simulink model "pd_controller"  (R2022a)
settings: Solver=VariableStepAuto  StartTime=0.0  StopTime=10.0  RelTol=1e-3
settings Model: Creator=Laptop-Academy.com  LastModifiedBy=Laptop-Academy.com

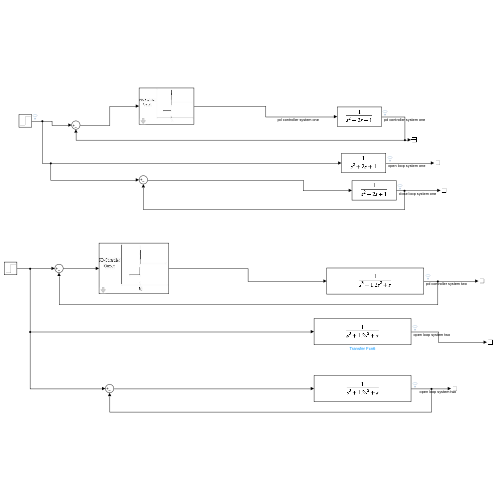
[thumbnail: Simulink's stored preview of the top-level diagram]
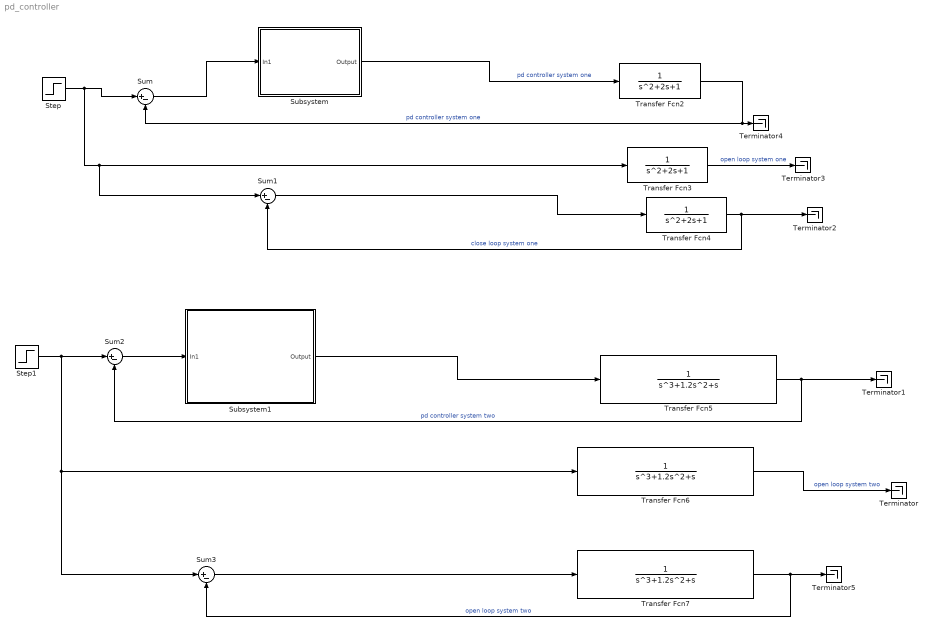
== system pd_controller ==
  Step : Step  SampleTime=0
  Step1 : Step  SampleTime=0
  Subsystem : Subsystem  mask{p=0, d=0}
      mask prompts: p "propotional gain (p)"; d "derivative gain (d)"
      mask Display: image("F:\os_academy_labs\pid_controller\media\pd.jpg")
  Subsystem1 : Subsystem  mask{p=0, d=0}
      mask prompts: p "proportional gain (p)"; d "derivartive gain (d)"
      mask Display: image("F:\os_academy_labs\pid_controller\media\pd.jpg")
  Sum{,1..3} (4 alike) : Sum  Inputs=|+-
  Terminator{,1..5} (6 alike) : Terminator
  Transfer Fcn2 : TransferFcn
  Transfer Fcn3 : TransferFcn
  Transfer Fcn4 : TransferFcn
  Transfer Fcn5 : TransferFcn  Denominator=[1 1.2 1 0]
  Transfer Fcn6 : TransferFcn  Denominator=[1 1.2 1 0]
  Transfer Fcn7 : TransferFcn  Denominator=[1 1.2 1 0]
  wires:
  Subsystem1/1(Output) -> Transfer Fcn5/1
  Transfer Fcn4/1 -> Sum1/2, Terminator2/1  "close loop system one"
  Transfer Fcn3/1 -> Terminator3/1  "open loop system one"
  Transfer Fcn2/1 -> Sum/2, Terminator4/1  "pd controller system one"
  Transfer Fcn6/1 -> Terminator/1  "open loop system two"
  Transfer Fcn7/1 -> Sum3/2, Terminator5/1  "open loop system two"
  Subsystem/1(Output) -> Transfer Fcn2/1  "pd controller system one"
  Transfer Fcn5/1 -> Sum2/2, Terminator1/1  "pd controller system two"
  Sum/1 -> Subsystem/1(In1)
  Step/1 -> Sum1/1, Transfer Fcn3/1, Sum/1
  Sum1/1 -> Transfer Fcn4/1
  Sum2/1 -> Subsystem1/1(In1)
  Step1/1 -> Sum3/1, Transfer Fcn6/1, Sum2/1
  Sum3/1 -> Transfer Fcn7/1

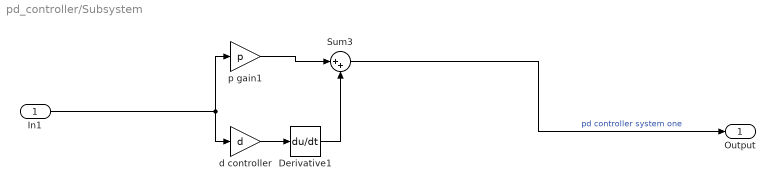
== system pd_controller/Subsystem ==
  In1 : Inport
  Derivative1 : Derivative
  Sum3 : Sum  Inputs=|++
  d controller : Gain  Gain=d
  p gain1 : Gain  Gain=p
  Output : Outport
  wires:
  Sum3/1 -> Output/1  "pd controller system one"
  In1/1 -> d controller/1, p gain1/1
  Derivative1/1 -> Sum3/2
  p gain1/1 -> Sum3/1
  d controller/1 -> Derivative1/1

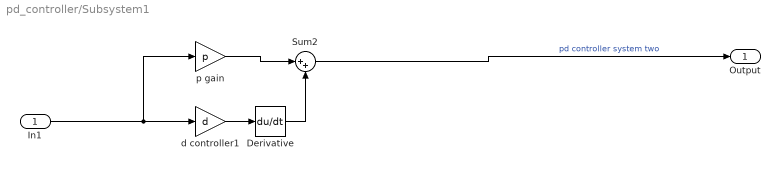
== system pd_controller/Subsystem1 ==
  In1 : Inport
  Derivative : Derivative
  Sum2 : Sum  Inputs=|++
  d controller1 : Gain  Gain=d
  p gain : Gain  Gain=p
  Output : Outport
  wires:
  Sum2/1 -> Output/1  "pd controller system two"
  In1/1 -> p gain/1, d controller1/1
  d controller1/1 -> Derivative/1
  p gain/1 -> Sum2/1
  Derivative/1 -> Sum2/2
